simulink model "Tank_Modell_Student"  (R2015b)
settings: Solver=ode45  StartTime=0.0  StopTime=400  MaxStep=1e-1  RelTol=1e-3
InitFcn:
  | set_parameter
StopFcn:
  | animation(h1_out,h2_out,q12_out,a1_out,a2_out,z1_out,anim_on,video_on);
values from neighbouring files (symbols this model uses):
  parSys =     [parameter_08.mat]
undefined symbols (not defined in the file or in its folder): parSollwertfilter
settings Model: Creator=Wolfgang Kemmetmüller  LastModifiedBy=danielhauer
settings DataIOCC: SaveFormat=Array
settings OptimizationCC: ExpressionDepthLimit=2147483647  InitFltsAndDblsToZero=on
settings DebuggingCC: SaveWithParameterizedLinksMsg=none  UnderspecifiedInitializationDetection=Classic  MergeDetectMultiDrivingBlocksExec=none  SolverPrmCheckMsg=warning  StateNameClashWarn=warning
settings HardwareCC: ProdBitPerPointer=32  ProdLargestAtomicFloat=None  ProdIntDivRoundTo=Undefined  ProdEndianess=Unspecified  ProdWordSize=32  ProdHWDeviceType=32-bit Generic
settings SFSimCC: SimParseCustomCode=off
settings GRTTargetCC: GeneratePreprocessorConditionals=Disable all  CombineOutputUpdateFcns=off  GRTInterface=on
settings ConfigComp: CovModelRefEnable=Off

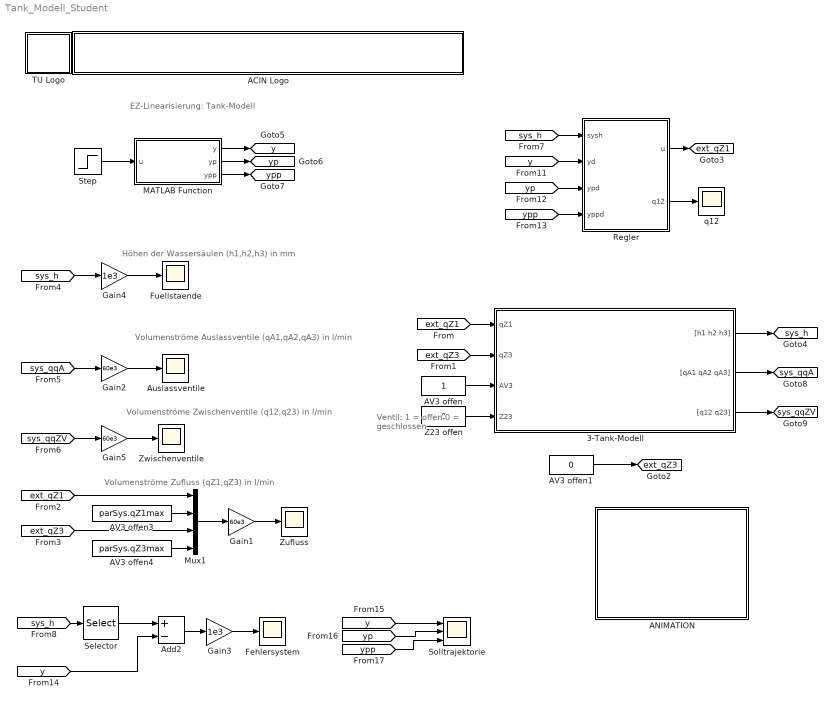
== system Tank_Modell_Student ==
  note: EZ-Linearisierung: Tank-Modell
  note: Höhen der Wassersäulen (h1,h2,h3) in mm
  note: Volumenströme Auslassventile (qA1,qA2,qA3) in l/min
  note: Volumenströme Zwischenventile (q12,q23) in l/min
  note: Ventil:
      | 1 = offen
      | 0 = geschlossen
  note: Volumenströme Zufluss (qZ1,qZ3) in l/min
  3-Tank-Modell : Subsystem
      mask init:
      | S = get_param(gcb,'UserData');
      mask Display:
      | image(S.pic);
      | port_label('input', 1, 'qZ1');
      | port_label('input', 2, 'qZ3');
      | port_label('input', 3, 'AV3');
      | port_label('input', 4, 'Z23');
      | port_label('output', 1, '[h1 h2 h3]');
      | port_label('output', 2, '[qA1 qA2 qA3]');
      | port_label('output', 3, '[q12 q23]');
  ACIN Logo : Subsystem
      mask init:
      | s = get_param(gcb,'UserData');
      mask Display:
      | image(s.logo,[0 0 439 45]);
      | %axis image
  ANIMATION : Subsystem
      mask init:
      | S = get_param(gcb,'UserData');
      mask Display: image(imread('Fisch.jpg'));
  AV3 offen : Constant
  AV3 offen1 : Constant  Value=0
  AV3 offen3 : Constant  Value=parSys.qZ1max  SampleTime=parSys.Ta
  AV3 offen4 : Constant  Value=parSys.qZ3max  SampleTime=parSys.Ta
  Add2 : Sum  Inputs=+-
  Auslassventile : Scope
  Fehlersystem : Scope
  Fuellstaende : Scope
  Gain1 : Gain  Gain=60e3
  Gain2 : Gain  Gain=60e3
  Gain3 : Gain  Gain=1e3
  Gain4 : Gain  Gain=1e3
  Gain5 : Gain  Gain=60e3
  MATLAB Function : MATLAB Function  TreatAsAtomicUnit=on  SystemSampleTime=parSollwertfilter.Ta
  Mux1 : Mux
  "Regler " : MATLAB Function  TreatAsAtomicUnit=on
  Selector : Selector  InputPortWidth=3  IndexOptions=Index vector (dialog)  Indices=[2]  OutputSizes=1
  Solltrajektorie : Scope  NumInputPorts=3
  Step : Step  Before=0.1  After=0.2  SampleTime=0
  TU Logo : Subsystem
      mask init:
      | s = get_param(gcb,'UserData');
      mask Display: image(s.logo,[0 0 45 45]);
  Z23 offen : Constant  Value=0
  Zufluss : Scope
  Zwischenventile : Scope
  q12 : Scope
  tag scope: ext_qZ1=global, ext_qZ3=global, sys_h=global, sys_qqA=global, sys_qqZV=global, y=global, yp=global, ypp=global
  wires:
  [sys_qqA] -> Gain2/1
  [sys_qqZV] -> Gain5/1
  [sys_h] -> Gain4/1
  3-Tank-Modell/1("[h1 h2 h3]") -> [sys_h]
  3-Tank-Modell/3("[q12 q23]") -> [sys_qqZV]
  3-Tank-Modell/2("[qA1 qA2 qA3]") -> [sys_qqA]
  AV3 offen/1 -> 3-Tank-Modell/3(AV3)
  Z23 offen/1 -> 3-Tank-Modell/4(Z23)
  [ext_qZ1] -> 3-Tank-Modell/1(qZ1)
  [ext_qZ3] -> 3-Tank-Modell/2(qZ3)
  [ext_qZ1] -> Mux1/1
  [ext_qZ3] -> Mux1/3
  AV3 offen3/1 -> Mux1/2
  AV3 offen4/1 -> Mux1/4
  Gain5/1 -> Zwischenventile/1
  Gain2/1 -> Auslassventile/1
  Gain4/1 -> Fuellstaende/1
  Mux1/1 -> Gain1/1
  Gain1/1 -> Zufluss/1
  AV3 offen1/1 -> [ext_qZ3]
  "Regler "/1(u) -> [ext_qZ1]
  Step/1 -> MATLAB Function/1(u)
  [sys_h] -> "Regler "/1(sysh)
  [sys_h] -> Selector/1
  Selector/1 -> Add2/1
  "Regler "/2(q12) -> q12/1
  MATLAB Function/3(ypp) -> [ypp]
  MATLAB Function/2(yp) -> [yp]
  MATLAB Function/1(y) -> [y]
  [y] -> "Regler "/2(yd)
  [yp] -> "Regler "/3(ypd)
  [ypp] -> "Regler "/4(yppd)
  [y] -> Add2/2
  [y] -> Solltrajektorie/1
  [yp] -> Solltrajektorie/2
  [ypp] -> Solltrajektorie/3
  Add2/1 -> Gain3/1
  Gain3/1 -> Fehlersystem/1

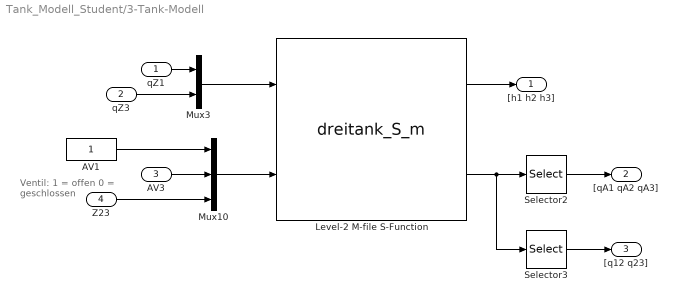
== system Tank_Modell_Student/3-Tank-Modell ==
  note: Ventil:
      | 1 = offen
      | 0 = geschlossen
  qZ1 : Inport
  qZ3 : Inport  Port=2
  AV3 : Inport  Port=3
  Z23 : Inport  Port=4
  AV1 : Constant
  Level-2 M-file S-Function : M-S-Function  FunctionName=dreitank_S_m  Parameters=Atank, rho, eta, g, alphaA1, DA1, alphaA2, A2, alphaA3, DA3, alpha12_0, A12, Dh12, lambdac12, alpha23_0, D23, lambdac23, hmin, h1_0, h2_0, h3_0, qZ1max, qZ3max, flaglimqZ, h_max, h_min  mask{Atank=parSys.Atank, rho=parSys.rho, eta=parSys.eta, g=parSys.g, alphaA1=parSys.alphaA1, DA1=parSys.DA1, alphaA2=parSys.alphaA2, A2=parSys.A2, alphaA3=parSys.alphaA3, DA3=parSys.DA3, alpha12_0=parSys.alpha12_0, A12=parSys.A12, Dh12=parSys.Dh12, lambdac12=parSys.lambdac12, alpha23_0=parSys.alpha23_0, D23=parSys.D23, lambdac23=parSys.lambdac23, hmin=parSys.hmin, h1_0=parSys.h1_0, h2_0=parSys.h2_0, h3_0=parSys.h3_0, qZ1max=parSys.qZ1max, qZ3max=parSys.qZ3max, h_max=parSys.hmax, h_min=parSys.hmin, flaglimqZ=off}
      mask prompts: Atank "Grundfläche Tank (Atank)"; rho "Dichte Wasser (rho)"; eta "Viskosität Wasser (eta)"; g "Gravitationskonstante (g)"; alphaA1 "Kontraktionskoeffizient AV1 (alphaA1)"; DA1 "Durchmesser AV1 (DA1)"; alphaA2 "Kontraktionskoeffizient AV2 (alphaA2)"; A2 "Querschnittsfläche AV2 (A2)"; alphaA3 "Kontraktionskoeffizient AV3 (alphaA3)"; DA3 "Durchmesser A3 (DA3)"; alpha12_0 "Kontraktionskoeffizient ZV12 (alpha12_0)"; A12 "Querschnittsfläche ZV12 (A12)"; Dh12 "hydraulischer Durchmesser ZV12 (Dh12)"; lambdac12 "kritische Fließzahl ZV12 (lambdac12)"; alpha23_0 "Kontraktionskoeffizient ZV23 (alpha23_0)"; D23 "Durchmesser ZV23 (D23)"; lambdac23 "kritische Fließzahl ZV23 (lambdac23)"; hmin "minimale Füllhöhe (hmin)"; h1_0 "Anfangsbedingung h1 (h1_0)"; h2_0 "Anfangsbedingung h2 (h2_0)"; h3_0 "Anfangsbedingung h3 (h3_0)"; qZ1max "maximaler Zufluss Z1 (qZ1max)"; qZ3max "maximaler Zufluss Z3 (qZ3max)"; h_max "Maximale Füllhöhe"; h_min "Minimale Füllhöhe"; flaglimqZ "Beschränkung der Zuflüsse ein"
      mask Display:
      | port_label('input',1,'Zulaufvolumenströme')
      | port_label('input',2,'Zustand Ventile')
      | 
      | port_label('output',1,'Zustände')
      | port_label('output',2,'Volumenströme')
  Mux10 : Mux  Inputs=3
  Mux3 : Mux  Inputs=2
  Selector2 : Selector  InputPortWidth=5  IndexOptions=Index vector (dialog)  Indices=[1 2 3]  OutputSizes=1
  Selector3 : Selector  InputPortWidth=5  IndexOptions=Index vector (dialog)  Indices=[4 5]  OutputSizes=1
  "[h1 h2 h3]" : Outport
  "[qA1 qA2 qA3]" : Outport  Port=2
  "[q12 q23]" : Outport  Port=3
  wires:
  AV1/1 -> Mux10/1
  Mux3/1 -> Level-2 M-file S-Function/1
  Mux10/1 -> Level-2 M-file S-Function/2
  qZ1/1 -> Mux3/1
  Level-2 M-file S-Function/1 -> "[h1 h2 h3]"/1
  qZ3/1 -> Mux3/2
  Level-2 M-file S-Function/2 -> Selector2/1, Selector3/1
  Selector2/1 -> "[qA1 qA2 qA3]"/1
  Selector3/1 -> "[q12 q23]"/1
  Z23/1 -> Mux10/3
  AV3/1 -> Mux10/2

== system Tank_Modell_Student/ACIN Logo ==

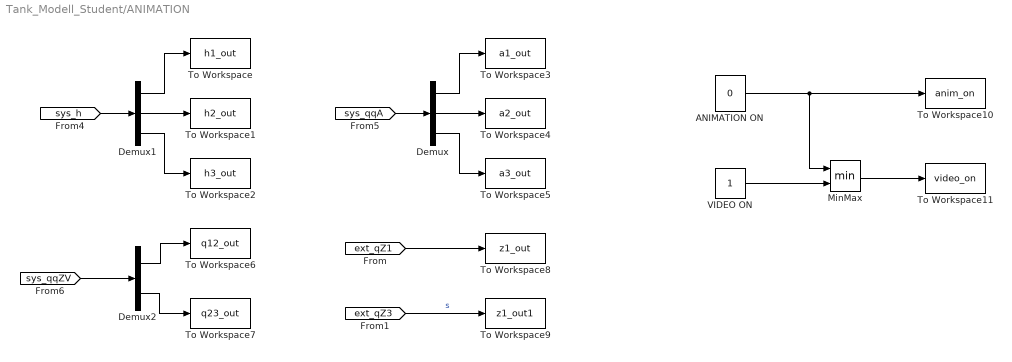
== system Tank_Modell_Student/ANIMATION ==
  ANIMATION ON : Constant  Value=0
  Demux : Demux  Outputs=3
  Demux1 : Demux  Outputs=3
  Demux2 : Demux  Outputs=2
  MinMax : MinMax  Inputs=2
  To Workspace : ToWorkspace  VariableName=h1_out  SampleTime=parSys.Ta
  To Workspace1 : ToWorkspace  VariableName=h2_out  SampleTime=parSys.Ta
  To Workspace10 : ToWorkspace  VariableName=anim_on  SampleTime=50
  To Workspace11 : ToWorkspace  VariableName=video_on  SampleTime=50
  To Workspace2 : ToWorkspace  VariableName=h3_out  SampleTime=parSys.Ta
  To Workspace3 : ToWorkspace  VariableName=a1_out  SampleTime=parSys.Ta
  To Workspace4 : ToWorkspace  VariableName=a2_out  SampleTime=parSys.Ta
  To Workspace5 : ToWorkspace  VariableName=a3_out  SampleTime=parSys.Ta
  To Workspace6 : ToWorkspace  VariableName=q12_out  SampleTime=parSys.Ta
  To Workspace7 : ToWorkspace  VariableName=q23_out  SampleTime=parSys.Ta
  To Workspace8 : ToWorkspace  VariableName=z1_out  SampleTime=parSys.Ta
  To Workspace9 : ToWorkspace  VariableName=z1_out1  SampleTime=parSys.Ta
  VIDEO ON : Constant
  wires:
  [sys_qqA] -> Demux/1
  Demux/1 -> To Workspace3/1
  Demux/2 -> To Workspace4/1
  Demux/3 -> To Workspace5/1
  [sys_h] -> Demux1/1
  Demux1/1 -> To Workspace/1
  Demux1/2 -> To Workspace1/1
  Demux1/3 -> To Workspace2/1
  Demux2/1 -> To Workspace6/1
  Demux2/2 -> To Workspace7/1
  [sys_qqZV] -> Demux2/1
  [ext_qZ1] -> To Workspace8/1
  [ext_qZ3] -> To Workspace9/1  "s"
  ANIMATION ON/1 -> MinMax/1, To Workspace10/1
  MinMax/1 -> To Workspace11/1
  VIDEO ON/1 -> MinMax/2

== system Tank_Modell_Student/TU Logo ==

== matlab function Tank_Modell_Student/MATLAB Function ==
  settings: updateMethod=DISCRETE  sampleTime=parSollwertfilter.Ta
  data: u input; y output; yp output; ypp output; parSollwertfilter parameter; parSys parameter
function [y,yp,ypp] = sollwertfilter(u, parSollwertfilter, parSys)
persistent x;

u = u-parSys.h2_0; % Anfangswert abziehen

a=parSollwertfilter.a;
b=parSollwertfilter.b;
c=parSollwertfilter.c;
d=parSollwertfilter.d;

if(isempty(x))
    x0_Filter=parSollwertfilter.x0_Filter;
    x=x0_Filter;
end

yt=c*x+d*u;
y=yt(1)+parSys.h2_0; % Anfangswert wieder addieren
yp=yt(2);
ypp=yt(3);

x=a*x+b*u;

== matlab function Tank_Modell_Student/Regler  ==
  settings: updateMethod=DISCRETE  sampleTime=parSys.Ta
  data: u output; sysh input; parSys parameter; yd input; ypd input; yppd input; q12 output
function [u,q12]  = fcn(sysh, parSys, yd, ypd, yppd)

Atank = parSys.Atank;
rho = parSys.rho;
eta = parSys.eta;
g = parSys.g;
alphaA1 = parSys.alphaA1;
DA1 = parSys.DA1;
alphaA2 = parSys.alphaA2;
A2 = parSys.A2;
alphaA3 = parSys.alphaA3;
DA3 = parSys.DA3;
alpha12_0 = parSys.alpha12_0;
A12 = parSys.A12;
Dh12 = parSys.Dh12;
lambdac12 = parSys.lambdac12;
alpha23_0 = parSys.alpha23_0;
D23 = parSys.D23;
lambdac23 = parSys.lambdac23;
hmin = parSys.hmin;
hmax = parSys.hmax;
dh12min = parSys.dh12min;
a0 = parSys.a0;
a1 = parSys.a1;

h1=sysh(1);
h2=sysh(2);
qA1 = alphaA1 * DA1 ^ 2 * pi * sqrt(0.2e1) * sqrt(g) * sqrt(h1) / 0.4e1;
qA2 = alphaA2 * A2 * sqrt(0.2e1) * sqrt(g) * sqrt(h2);

dqA2_dh2 = alphaA2 * A2 * sqrt(0.2e1) * sqrt(g) * h2 ^ (-0.1e1 / 0.2e1) / 0.2e1;

if abs(h1-h2) > dh12min
    dq12_dh1 = 0.2e1 * alpha12_0 * Dh12 * rho / eta * g / lambdac12 * (0.1e1 - tanh(0.2e1 * Dh12 * rho / eta * sqrt(0.2e1) * sqrt(g) * sqrt(abs(h1 - h2)) / lambdac12) ^ 2) * A12 + alpha12_0 * tanh(0.2e1 * Dh12 * rho / eta * sqrt(0.2e1) * sqrt(g) * sqrt(abs(h1 - h2)) / lambdac12) * A12 * sqrt(0.2e1) * sqrt(g) * (abs(h1 - h2) ^ (-0.1e1 / 0.2e1)) / 0.2e1;
    dq12_dh2 = -0.2e1 * alpha12_0 * Dh12 * rho / eta * g / lambdac12 * (0.1e1 - tanh(0.2e1 * Dh12 * rho / eta * sqrt(0.2e1) * sqrt(g) * sqrt(abs(h1 - h2)) / lambdac12) ^ 2) * A12 - alpha12_0 * tanh(0.2e1 * Dh12 * rho / eta * sqrt(0.2e1) * sqrt(g) * sqrt(abs(h1 - h2)) / lambdac12) * A12 * sqrt(0.2e1) * sqrt(g) * (abs(h1 - h2) ^ (-0.1e1 / 0.2e1)) / 0.2e1;
else
    %Linearisierung
    dq12_dh1 = parSys.d_dh1 + parSys.k_dh1*abs(h1-h2);
    dq12_dh2 = parSys.d_dh2 + parSys.k_dh2*abs(h1-h2);
end
q12 = alpha12_0 * tanh(0.2e1 * Dh12 * rho / eta * sqrt(0.2e1) * sqrt(g) * sqrt(abs(h1 - h2)) / lambdac12) * A12 * sqrt(0.2e1) * sqrt(g) * sqrt(abs(h1 - h2)) * sign((h1 - h2));

u = 0.1e1 / dq12_dh1 * Atank ^ 2 * (yppd - dq12_dh1 / Atank ^ 2 * (-q12 - qA1) - (dq12_dh2 - dqA2_dh2) / Atank ^ 2 * (q12 - qA2) - a0 * (h2 - yd) - a1 * ((q12 - qA2) / Atank - ypd));
